simulink model "SOFC_meca"  (R2021a)
settings: Solver=VariableStepAuto  StartTime=0.0  StopTime=NaN  RelTol=1e-3
undefined symbols (not defined in the file or in its folder): p
settings Model: Creator=djoroya  LastModifiedBy=djoroya

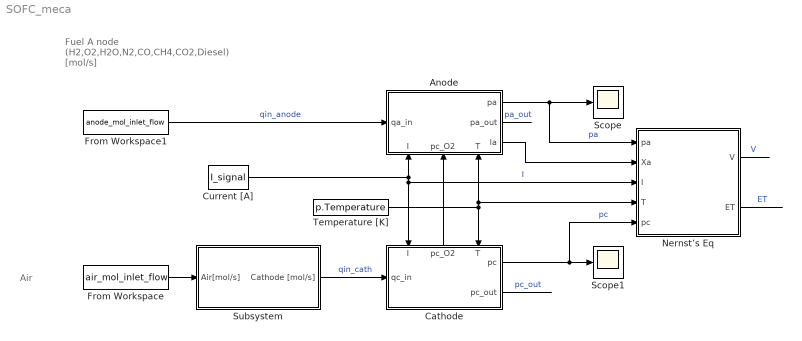
== system SOFC_meca ==
  note: Fuel
      | A node
      | (H2,O2,H2O,N2,CO,CH4,CO2,Diesel)
      | [mol/s]
  note: Air
  Anode : Subsystem
      settings: PortSchema="{\"entries\":[{\"content\":{\"sides\":[{\"content\":{\"connectorIds\":[\"In1\"]},\"type\":\"ConnectorPlacement.EquallySpacedRectSide\",\"uuid\":\"1d27f661-9cb9-482d-ac43-89e84d52643b\"},{\"content\":{\"connectorIds\":[\"Out1\",\"Out2\",\"Out3\"],\"side\":\"RIGHT\"},\"type\":\"ConnectorPlacement.EquallySpacedRectSide\",\"uuid\":\"62ac897d-5819-4e9c-a19f-e210851aefa2\"},{\"content\":{\"connectorIds\":[],\"side\":\"TOP\"},\"type\":\"ConnectorPlacement.EquallySpacedRectSide\",\"uuid\":\"1380e9d4-c5ac-42ce-b6fc-00336cc8edba\"},{\"content\":{\"connectorIds\":[\"In2\",\"In3\",\"In4\"],\"side\":\"BOTTOM\"},\"type\":\"ConnectorPlacement.EquallySpacedRectSide\",\"uuid\":\"0e36fd1a-38eb-48cb-8834-06d558b43614\"}]},\"type\":\"ConnectorPlacement.EquallySpacedConnector\",\"uuid\":\"79a72313-dbdc-4de5-b88f-787bafe984c7\"}],\"packageUris\":[\"http://schema.mathworks.com/mf0/Connector/R2020b\"],\"version\":\"1.0\"}"
  Cathode : Subsystem
      settings: PortSchema="{\"entries\":[{\"content\":{\"sides\":[{\"content\":{\"connectorIds\":[\"In1\"]},\"type\":\"ConnectorPlacement.EquallySpacedRectSide\",\"uuid\":\"1d27f661-9cb9-482d-ac43-89e84d52643b\"},{\"content\":{\"connectorIds\":[\"Out1\",\"Out2\"],\"side\":\"RIGHT\"},\"type\":\"ConnectorPlacement.EquallySpacedRectSide\",\"uuid\":\"62ac897d-5819-4e9c-a19f-e210851aefa2\"},{\"content\":{\"connectorIds\":[\"In2\",\"Out3\",\"In3\"],\"side\":\"TOP\"},\"type\":\"ConnectorPlacement.EquallySpacedRectSide\",\"uuid\":\"1380e9d4-c5ac-42ce-b6fc-00336cc8edba\"}]},\"type\":\"ConnectorPlacement.EquallySpacedConnector\",\"uuid\":\"79a72313-dbdc-4de5-b88f-787bafe984c7\"}],\"packageUris\":[\"http://schema.mathworks.com/mf0/Connector/R2020b\"],\"version\":\"1.0\"}"
  Current [A] : FromWorkspace  VariableName=I_signal
  From Workspace : FromWorkspace  VariableName=air_mol_inlet_flow
  From Workspace1 : FromWorkspace  VariableName=anode_mol_inlet_flow
  "Nernst’s Eq " : Subsystem
  Scope : Scope
  Scope1 : Scope
  Subsystem : Subsystem
  Temperature [K] : Constant  Value=p.Temperature
  wires:
  From Workspace/1 -> Subsystem/1(Air[mol/s])
  From Workspace1/1 -> Anode/1(qa_in)  "qin_anode"
  Subsystem/1(Cathode [mol/s]) -> Cathode/1(qc_in)  "qin_cath"
  Temperature [K]/1 -> "Nernst’s Eq "/4(T), Anode/4(T), Cathode/3(T)
  Anode/1(pa) -> "Nernst’s Eq "/1(pa), Scope/1  "pa"
  Anode/2(pa_out) -> ?  "pa_out"
  Cathode/1(pc) -> "Nernst’s Eq "/5(pc), Scope1/1  "pc"
  Cathode/2(pc_out) -> ?  "pc_out"
  Current [A]/1 -> Cathode/2(I), "Nernst’s Eq "/3(I), Anode/2(I)  "I"
  "Nernst’s Eq "/1(V) -> ?  "V"
  Anode/3(la) -> "Nernst’s Eq "/2(Xa)
  Cathode/3(pc_O2) -> Anode/3(pc_O2)
  "Nernst’s Eq "/2(ET) -> ?  "ET"

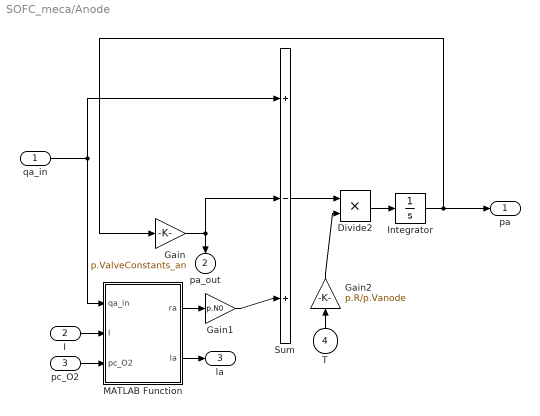
== system SOFC_meca/Anode ==
  qa_in : Inport
  I : Inport  Port=2
  pc_O2 : Inport  Port=3
  T : Inport  Port=4
  Divide2 : Product  Inputs=**
  Gain : Gain  Gain=p.ValveConstants_an
  Gain1 : Gain  Gain=p.N0
  Gain2 : Gain  Gain=p.R/p.Vanode
  Integrator : Integrator
  MATLAB Function : MATLAB Function  TreatAsAtomicUnit=on
  Sum : Sum  Inputs=|+-+
  pa : Outport
  pa_out : Outport  Port=2
  la : Outport  Port=3
  wires:
  Sum/1 -> Divide2/1
  Integrator/1 -> pa/1, Gain/1
  Gain2/1 -> Divide2/2
  qa_in/1 -> Sum/1, MATLAB Function/1(qa_in)
  Divide2/1 -> Integrator/1
  Gain/1 -> pa_out/1, Sum/2
  I/1 -> MATLAB Function/2(I)
  T/1 -> Gain2/1
  MATLAB Function/2(la) -> la/1
  pc_O2/1 -> MATLAB Function/3(pc_O2)
  MATLAB Function/1(ra) -> Gain1/1
  Gain1/1 -> Sum/3

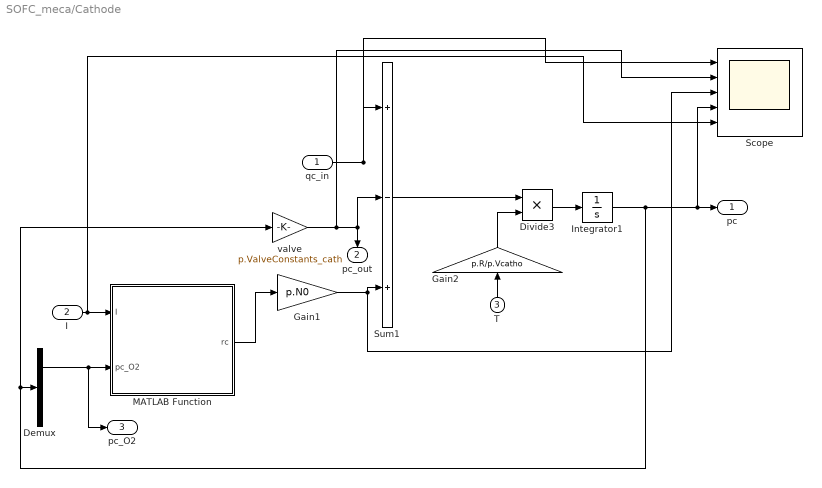
== system SOFC_meca/Cathode ==
  qc_in : Inport
  I : Inport  Port=2
  T : Inport  Port=3
  Demux : Demux  Outputs=7
  Divide3 : Product  Inputs=**
  Gain1 : Gain  Gain=p.N0
  Gain2 : Gain  Gain=p.R/p.Vcatho
  Integrator1 : Integrator
  MATLAB Function : MATLAB Function  TreatAsAtomicUnit=on
  Scope : Scope  NumInputPorts=5
  Sum1 : Sum  Inputs=|+-+
  valve : Gain  Gain=p.ValveConstants_cath
  pc : Outport
  pc_out : Outport  Port=2
  pc_O2 : Outport  Port=3
  wires:
  Sum1/1 -> Divide3/1
  Integrator1/1 -> valve/1, Demux/1, Scope/4, pc/1
  Divide3/1 -> Integrator1/1
  qc_in/1 -> Scope/1, Sum1/1
  Gain2/1 -> Divide3/2
  T/1 -> Gain2/1
  valve/1 -> Scope/2, pc_out/1, Sum1/2
  I/1 -> Scope/5, MATLAB Function/1(I)
  Demux/2 -> pc_O2/1, MATLAB Function/2(pc_O2)
  MATLAB Function/1(rc) -> Gain1/1
  Gain1/1 -> Scope/3, Sum1/3

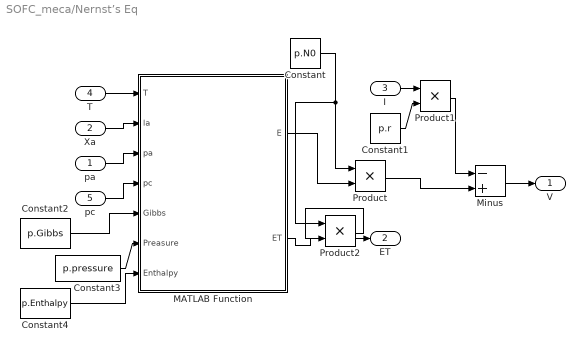
== system SOFC_meca/Nernst’s Eq  ==
  pa : Inport
  Xa : Inport  Port=2
  I : Inport  Port=3
  T : Inport  Port=4
  pc : Inport  Port=5
  Constant : Constant  Value=p.N0
  Constant1 : Constant  Value=p.r
  Constant2 : Constant  Value=p.Gibbs  OutDataTypeStr=Bus:slBus1
  Constant3 : Constant  Value=p.pressure
  Constant4 : Constant  Value=p.Enthalpy  OutDataTypeStr=Bus:slBus1
  MATLAB Function : MATLAB Function  TreatAsAtomicUnit=on
  Minus : Sum  Inputs=-+
  Product : Product
  Product1 : Product
  Product2 : Product
  V : Outport
  ET : Outport  Port=2
  wires:
  MATLAB Function/1(E) -> Product/2
  Constant/1 -> Product2/1, Product/1
  I/1 -> Product1/1
  Constant1/1 -> Product1/2
  Product/1 -> Minus/2
  Minus/1 -> V/1
  Product1/1 -> Minus/1
  pa/1 -> MATLAB Function/3(pa)
  pc/1 -> MATLAB Function/4(pc)
  Constant2/1 -> MATLAB Function/5(Gibbs)
  T/1 -> MATLAB Function/1(T)
  Xa/1 -> MATLAB Function/2(la)
  Constant3/1 -> MATLAB Function/6(Preasure)
  Constant4/1 -> MATLAB Function/7(Enthalpy)
  Product2/1 -> ET/1
  MATLAB Function/2(ET) -> Product2/2

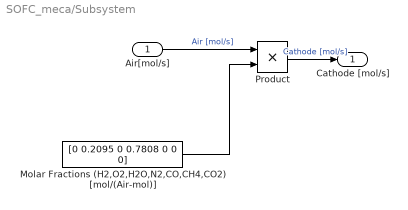
== system SOFC_meca/Subsystem ==
  Air[mol/s] : Inport
  Molar Fractions (H2,O2,H2O,N2,CO,CH4,CO2) [mol/(Air-mol)] : Constant  Value=[0 0.2095 0 0.7808 0 0 0]
  Product : Product
  Cathode [mol/s] : Outport
  wires:
  Air[mol/s]/1 -> Product/1  "Air [mol/s]"
  Product/1 -> Cathode [mol/s]/1  "Cathode [mol/s]"
  Molar Fractions (H2,O2,H2O,N2,CO,CH4,CO2) [mol/(Air-mol)]/1 -> Product/2

== matlab function SOFC_meca/Cathode/MATLAB Function ==
  data: rc output; I input; pc_O2 input
function rc = fcn(I,pc_O2)

%l = qc_in/sum(qc_in);

% l_H2  = l(1);
% l_O2  = l(2);
% l_H2O = l(3);
% l_N2  = l(4);
% l_CO  = l(5);
% l_CH4 = l(6);
% l_CO2 = l(7);
%
% alpha_H_2 = l_H2;
% alpha_CO  = l_CO;
% alpha_CH4 = l_CH4;
% alpha_O2  = 0.5*(l_H2+l_CO+4*l_CH4);
% beta_H2O  = l_H2 + 2*l_CH4;
% beta_CO2  = l_CO + 2*l_CH4;
%
F = 96485.3329; 

% r_H2  = -alpha_H_2*I;
% r_CO  = -alpha_CO*I;
% r_CH4 = -alpha_CH4*I;
% r_H20 = beta_H2O*I;
% r_CO2 = beta_CO2*I;
if pc_O2 <= 0
    r_O2  = 0;
else
    r_O2  = I/(4*F);
end

rc = [0 -r_O2 0 0 0 0 0]';

== matlab function SOFC_meca/Anode/MATLAB Function ==
  data: qa_in input; ra output; I input; la output; pc_O2 input
function [ra,la] = fcn(qa_in,I,pc_O2)

la = qa_in/sum(qa_in);

l_H2  = la(1);
%l_O2  = l(2);
%l_H2O = l(3);
%l_N2  = l(4);
l_CO  = la(5);
l_CH4 = la(6);
%l_CO2 = l(7);
%
alpha_H2 = l_H2;
alpha_CO  = l_CO;
alpha_CH4 = l_CH4;
%alpha_O2  = 0.5*(l_H2+l_CO+4*l_CH4);
beta_H2O  = l_H2 + 2*l_CH4;
beta_CO2  = l_CO + l_CH4;
%
F = 96485.3329; 
ne = 2*(l_H2 + l_CO + 4*l_CH4);
I = I/(F*ne);

r_H2  = -alpha_H2*I;
r_CO  = -alpha_CO*I;
r_CH4 = -alpha_CH4*I;
r_H20 = beta_H2O*I;
r_CO2 = beta_CO2*I;
%
ra = [r_H2 0 r_H20 0 r_CO r_CH4 r_CO2]';

if pc_O2 <= 0
    ra  = 0*ra;
end

== matlab function SOFC_meca/Nernst’s Eq /MATLAB Function ==
  data: T input; la input; pa input; E output; pc input; Gibbs input; Preasure input; Enthalpy input; ET output
function [E,ET]= fcn(T, la,pa,pc,Gibbs,Preasure, Enthalpy)
%

l_H2  = la(1);
l_CO  = la(5);
l_CH4 = la(6);
%
alpha_H2 = l_H2;
alpha_CO  = l_CO;
alpha_CH4 = l_CH4;
alpha_O2  = 0.5*( l_H2 + l_CO + 4*l_CH4);
beta_H2O  = l_H2 + 2*l_CH4;
beta_CO2  = l_CO + l_CH4;

%
pa_H2 = pa(1);
pa_O2 = pa(2);
pa_H2O= pa(3);
pa_CO = pa(5);
pa_CH4= pa(6);
pa_CO2= pa(7);
%
pc_H2 = pc(1);
pc_O2 = pc(2);
pc_H2O= pc(3);
pc_N2 = pc(4);
pc_CO = pc(5);
pc_CH4= pc(6);
pc_CO2= pc(7);
%% 
F = 96485.3329; 
ne = 2*(l_H2 + l_CO + 4*l_CH4);
%%
G = alpha_H2*Gibbs.H2 + ...
    alpha_CO*Gibbs.CO + ...
    alpha_CH4*Gibbs.CH4 + ...
    alpha_O2*Gibbs.O2 + ...
    - beta_H2O*Gibbs.H2O + ...
    - beta_CO2*Gibbs.CO2;
%%
E0 = G/(F*ne); 

%%
R = 8.31446261815324;

ab =    [alpha_H2, ...
         alpha_CO, ...
         alpha_CH4, ...
         alpha_O2,  ...
         -beta_H2O, ...
         -beta_CO2];
     
pa_ab = [pa_H2, ...
         pa_CO, ...
         pa_CH4, ...
         pc_O2,  ...
         pa_H2O, ...
         pa_CO2];
     
log_ab = 0*ab;
iter = 0;
for ipa_ab = pa_ab
    iter = iter + 1;
    if ipa_ab > 0
       log_ab(iter) =  log(ipa_ab/Preasure);
    end
end

E = E0 + ((R*T)/(ne*F))*( sum(log_ab.*ab) );

%%
H = alpha_H2*Enthalpy.H2 + ...
    alpha_CO*Enthalpy.CO + ...
    alpha_CH4*Enthalpy.CH4 + ...
    alpha_O2*Enthalpy.O2 + ...
    - beta_H2O*Enthalpy.H2O + ...
    - beta_CO2*Enthalpy.CO2;
ET = H/(ne*F);
%
